simulink model "linmodel_eq1_discr3_lqr"  (R2019a)
settings: Solver=VariableStepAuto  StartTime=0.0  StopTime=30  RelTol=1e-3
InitFcn:
  | lin_discr_model
undefined symbols (not defined in the file): A_eq1_d, B_eq1_d, C_eq1_d, K1, L2, Ts
settings Model: Creator=jessi  LastModifiedBy=jessi

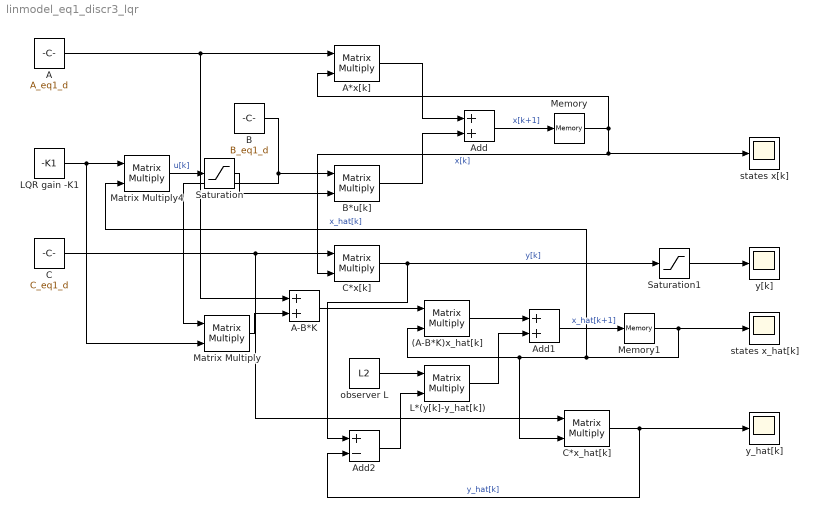
== system linmodel_eq1_discr3_lqr ==
  (A-B*K)x_hat[k] : Product  Multiplication=Matrix(*)
  A : Constant  Value=A_eq1_d  SampleTime=Ts
  A*x[k] : Product  Multiplication=Matrix(*)
  A-B*K : Sum
  Add : Sum
  Add1 : Sum
  Add2 : Sum  Inputs=+-
  B : Constant  Value=B_eq1_d  SampleTime=Ts
  B*u[k] : Product  Multiplication=Matrix(*)
  C : Constant  Value=C_eq1_d  SampleTime=Ts
  C*x[k] : Product  Multiplication=Matrix(*)
  C*x_hat[k] : Product  Multiplication=Matrix(*)
  L*(y[k]-y_hat[k]) : Product  Multiplication=Matrix(*)
  LQR gain -K1 : Constant  Value=-K1
  Matrix Multiply : Product  Multiplication=Matrix(*)
  Matrix Multiply4 : Product  Multiplication=Matrix(*)
  Memory : Memory  InitialCondition=[pi;0;0;0]
  Memory1 : Memory  InitialCondition=[pi;0;0;0]
  Saturation : Saturate  UpperLimit=10  LowerLimit=-10
  Saturation1 : Saturate  UpperLimit=2*pi  LowerLimit=-2*pi
  observer L : Constant  Value=L2  SampleTime=Ts
  states x[k] : Scope
  states x_hat[k] : Scope
  y[k] : Scope
  y_hat[k] : Scope
  wires:
  B/1 -> Matrix Multiply/1, B*u[k]/1
  A/1 -> A-B*K/1, A*x[k]/1
  A*x[k]/1 -> Add/1
  B*u[k]/1 -> Add/2
  Add/1 -> Memory/1  "x[k+1]"
  Memory/1 -> A*x[k]/2, states x[k]/1, C*x[k]/2  "x[k]"
  C/1 -> C*x_hat[k]/1, C*x[k]/1
  C*x[k]/1 -> Add2/1, Saturation1/1  "y[k]"
  A-B*K/1 -> (A-B*K)x_hat[k]/1
  (A-B*K)x_hat[k]/1 -> Add1/1
  L*(y[k]-y_hat[k])/1 -> Add1/2
  Add1/1 -> Memory1/1  "x_hat[k+1]"
  Memory1/1 -> states x_hat[k]/1, Matrix Multiply4/2, C*x_hat[k]/2, (A-B*K)x_hat[k]/2  "x_hat[k]"
  C*x_hat[k]/1 -> Add2/2, y_hat[k]/1  "y_hat[k]"
  LQR gain -K1/1 -> Matrix Multiply/2, Matrix Multiply4/1
  Matrix Multiply4/1 -> Saturation/1  "u[k]"
  Matrix Multiply/1 -> A-B*K/2
  observer L/1 -> L*(y[k]-y_hat[k])/1
  Add2/1 -> L*(y[k]-y_hat[k])/2
  Saturation/1 -> B*u[k]/2
  Saturation1/1 -> y[k]/1
